simulink model "rampa_23_10"  (R2020a)
settings: Solver=VariableStepAuto  StartTime=0.0  StopTime=10.0  RelTol=1e-3
undefined symbols (not defined in the file or in its folder): T
libraries: simulink x1
settings Model: Creator=jguil  LastModifiedBy=jguil

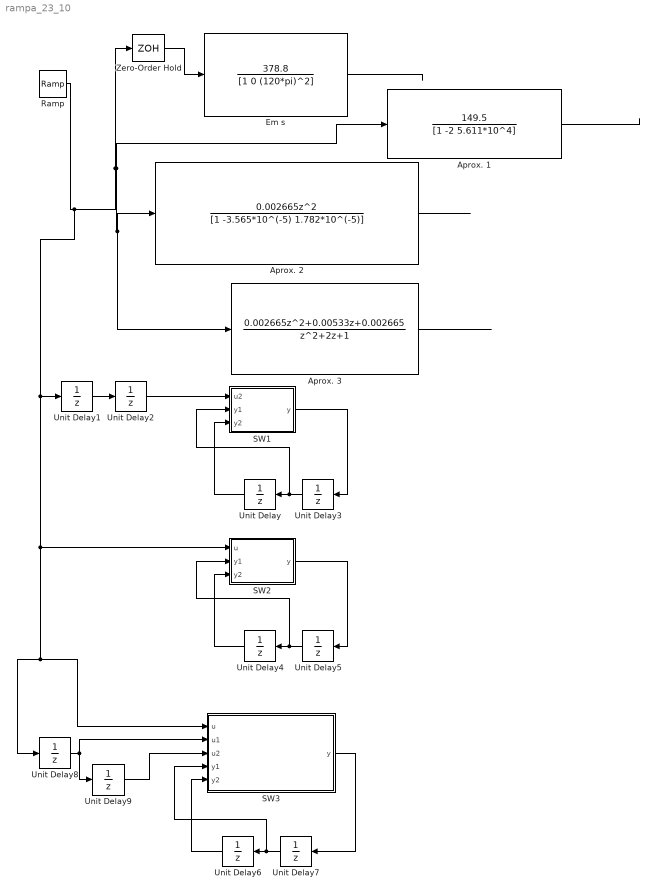
== system rampa_23_10 ==
  Aprox. 1 : DiscreteTransferFcn  Numerator=149.5  Denominator=[1 -2 5.611*10^4]  SampleTime=T
  Aprox. 2 : DiscreteTransferFcn  Numerator=[0.002665 0 0]  Denominator=[1 -3.565*10^(-5) 1.782*10^(-5)]  SampleTime=T
  Aprox. 3 : DiscreteTransferFcn  Numerator=[0.002665 0.00533 0.002665]  Denominator=[1 2 1]  SampleTime=T
  Em s : TransferFcn  Numerator=[378.8]  Denominator=[1 0 (120*pi)^2]
  Ramp : simulink/Sources/Ramp  slope=1  start=0  InitialOutput=0
  SW1 : MATLAB Function  TreatAsAtomicUnit=on
  SW2 : MATLAB Function  TreatAsAtomicUnit=on
  SW3 : MATLAB Function  TreatAsAtomicUnit=on
  Unit Delay{,1..9} (10 alike) : UnitDelay  SampleTime=T  HasFrameUpgradeWarning=on
  Zero-Order Hold : ZeroOrderHold  SampleTime=-1
  wires:
  Unit Delay4/1 -> SW2/3(y2)
  Unit Delay9/1 -> SW3/3(u2)
  Unit Delay5/1 -> SW2/2(y1), Unit Delay4/1
  Unit Delay6/1 -> SW3/5(y2)
  Unit Delay7/1 -> SW3/4(y1), Unit Delay6/1
  SW1/1(y) -> Unit Delay3/1
  Unit Delay/1 -> SW1/3(y2)
  Unit Delay1/1 -> Unit Delay2/1
  Ramp/1 -> Unit Delay8/1, SW3/1(u), SW2/1(u), Unit Delay1/1, Zero-Order Hold/1, Aprox. 3/1, Aprox. 2/1, Aprox. 1/1
  Em s/1 -> ?
  Unit Delay8/1 -> SW3/2(u1), Unit Delay9/1
  Aprox. 3/1 -> ?
  Unit Delay2/1 -> SW1/1(u2)
  Zero-Order Hold/1 -> Em s/1
  Aprox. 2/1 -> ?
  Aprox. 1/1 -> ?
  Unit Delay3/1 -> SW1/2(y1), Unit Delay/1
  SW3/1(y) -> Unit Delay7/1
  SW2/1(y) -> Unit Delay5/1

== matlab function rampa_23_10/SW2 ==
  data: u input; y output; y1 input; y2 input
function y = aprox2(u,y1,y2)
% y(n) = 3.565e(-5)*y(n-1) -1.782e(-5) *y(n-2)+0.002665*u(n)
y = 3.565*10^(-5)*y1 -1.782*10^(-5)*y2 +0.002665*u;

== matlab function rampa_23_10/SW1 ==
  data: u2 input; y output; y1 input; y2 input
function y = aprox1(u2,y1,y2)
% y(n) = 2*y(n-1) -5.611e4 *y(n-2)+149.5*u(n-2)
y = 2*y1-5.611*10^4*y2+149.5*u2;

== matlab function rampa_23_10/SW3 ==
  data: u input; y output; u1 input; u2 input; y1 input; y2 input
function y = aprox3(u,u1,u2,y1,y2)
% y(n) = -2*y(n-1) -y(n-2)+ 0.002665*u(n)+0.00533*u(n-1)+0.002665*u(n-2)
y = -2*y1-y2+0.002665*u+0.00533*u1+0.002665*u2;
